simulink model "harness"  (R2024b)
settings: Solver=ode45  StartTime=0.0  StopTime=100  FixedStep=1/10  RelTol=1e-3
InitFcn:
  | init_fn()
undefined symbols (not defined in the file): sigbuilder_block
libraries: simulink x9
settings Model: PacingRate=10  Creator=Jacopo Sini  LastModifiedBy=aayan
settings OptimizationCC: ReuseModelBlockBuffer=off
settings DebuggingCC: UnconnectedInputMsg=warning  UnconnectedOutputMsg=warning  UnconnectedLineMsg=warning
settings ModelReferenceCC: EnableRefExpFcnMdlSchedulingChecks=on
settings RTWCC: GPUComputeCapability=3.5  DLArmComputeVersion=19.05

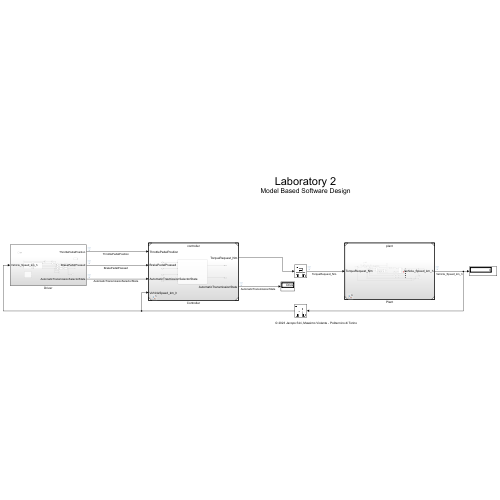
[thumbnail: Simulink's stored preview of the top-level diagram]
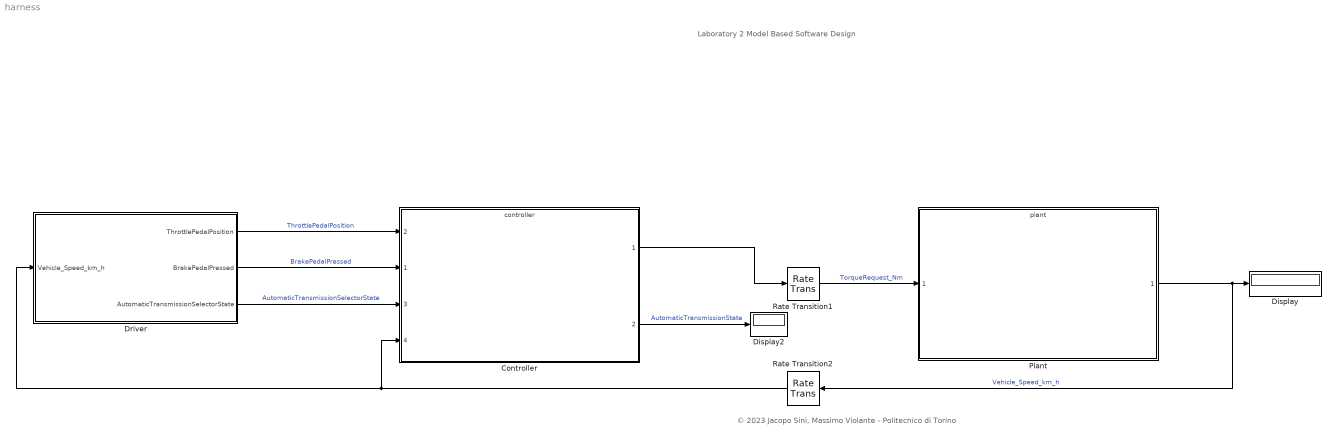
== system harness ==
  note: © 2023 Jacopo Sini, Massimo Violante - Politecnico di Torino
  note: Laboratory 2
      | Model Based Software Design
  Controller : ModelReference  ModelNameDialog=controller  SimulationMode=Normal  ModelReferenceVersion=7.15
      settings: PortSchema="{\"entries\":[{\"content\":{\"sides\":[{\"content\":{\"connectorIds\":[\"In2\",\"In1\",\"In3\",\"In4\"]},\"type\":\"ConnectorPlacement.EquallySpacedRectSide\",\"uuid\":\"5e260b81-e1ce-497c-8572-ac5c2182ee27\"},{\"content\":{\"connectorIds\":[\"Out1\",\"Out2\"],\"side\":\"RIGHT\"},\"type\":\"ConnectorPlacement.EquallySpacedRectSide\",\"uuid\":\"4325f63c-e453-4c79-ab01-1476da99aa25\"},{\"content\":{\"connectorIds\":[],\"side\":\"TOP\"},\"type\":\"ConnectorPlacement.EquallySpacedRectSide\",\"uuid\":\"dba88bac-0f95-4a98-ba3b-c40df5616f56\"}]},\"type\":\"ConnectorPlacement.EquallySpacedConnector\",\"uuid\":\"6943e10d-f3b0-4fd8-a142-b6b49e651f90\"}],\"packageUris\":[\"http://schema.mathworks.com/mf0/Connector/R2020b\"],\"version\":\"1.0\"}"
  Display : Display
  Display2 : Display
  Driver : Subsystem
  Plant : ModelReference  ModelNameDialog=plant  SimulationMode=Normal  ModelReferenceVersion=3.19
  Rate Transition1 : RateTransition
  Rate Transition2 : RateTransition
  wires:
  Plant/1 -> Rate Transition2/1, Display/1  "Vehicle_Speed_km_h"
  Controller/1 -> Rate Transition1/1
  Rate Transition2/1 -> Driver/1(Vehicle_Speed_km_h), Controller/4
  Controller/2 -> Display2/1  "AutomaticTransmissionState"
  Rate Transition1/1 -> Plant/1  "TorqueRequest_Nm"
  Driver/1(ThrottlePedalPosition) -> Controller/2  "ThrottlePedalPosition"
  Driver/2(BrakePedalPressed) -> Controller/1  "BrakePedalPressed"
  Driver/3(AutomaticTransmissionSelectorState) -> Controller/3  "AutomaticTransmissionSelectorState"

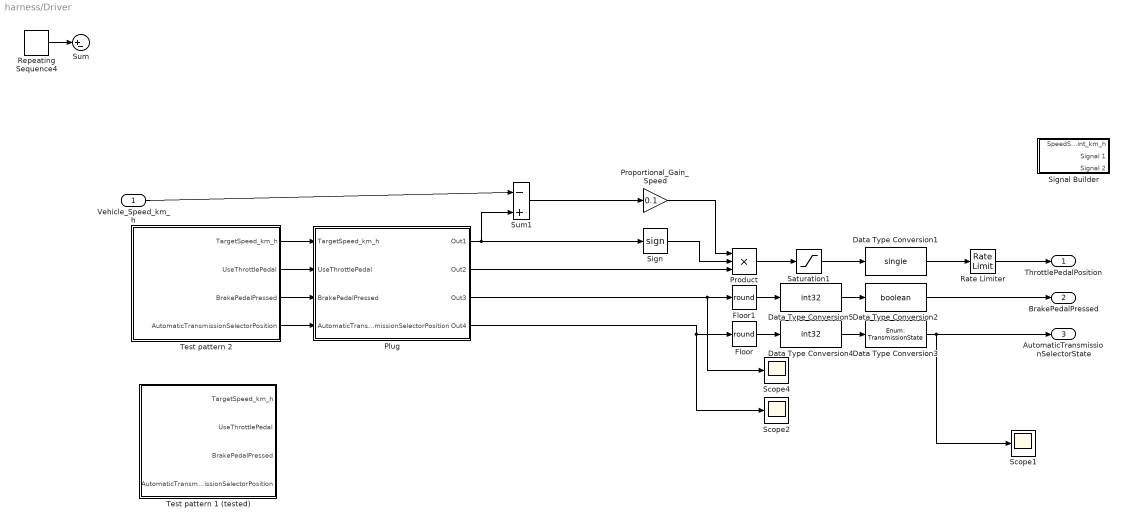
== system harness/Driver ==
  Vehicle_Speed_km_h : Inport
  Data Type Conversion1 : DataTypeConversion  OutDataTypeStr=single  SaturateOnIntegerOverflow=off  RndMeth=Floor  LockScale=on
  Data Type Conversion2 : DataTypeConversion  OutDataTypeStr=boolean  SaturateOnIntegerOverflow=off  RndMeth=Floor  LockScale=on
  Data Type Conversion3 : DataTypeConversion  OutDataTypeStr=Enum: TransmissionState  SaturateOnIntegerOverflow=off  RndMeth=Floor  LockScale=on
  Data Type Conversion4 : DataTypeConversion  OutDataTypeStr=int32  SaturateOnIntegerOverflow=off  RndMeth=Floor  LockScale=on
  Data Type Conversion5 : DataTypeConversion  OutDataTypeStr=int32  SaturateOnIntegerOverflow=off  RndMeth=Floor  LockScale=on
  Floor : Rounding  Operator=round
  Floor1 : Rounding  Operator=round
  Plug : Subsystem
  Product : Product  Inputs=3
  Proportional_Gain_Speed : Gain  Gain=0.1
  Rate Limiter : RateLimiter  RisingSlewLimit=0.5  SampleTimeMode=inherited
  Repeating Sequence4 : simulink/Sources/Repeating Sequence  rep_seq_t=[0 10 500]  rep_seq_y=[10 0 0]
  Saturation1 : Saturate  UpperLimit=1  LowerLimit=0
  Scope1 : Scope
  Scope2 : Scope
  Scope4 : Scope
  Sign : Signum
  Signal Builder : Subsystem  Tag=STV Subsys  LoadFcn=sigbuilder_block('load');  StartFcn=sigbuilder_block('start');  StopFcn=sigbuilder_block('stop');  ClipboardFcn=sigbuilder_block('clipboard');  mask(Sigbuilder block){tuvar=[0:10]}
      mask help: Simulink:masks:SigbuilderBlock_MD
      mask init:
      | if ~strcmp(get_param(bdroot(gcbh),'SimulationStatus'),'stopped') tuvar = sigbuilder_block('maskInit'); end
      settings: CopyFcn=sigbuilder_block('copy');  DeleteFcn=sigbuilder_block('delete');  ModelCloseFcn=sigbuilder_block('modelClose');  PreSaveFcn=sigbuilder_block('preSave');  PauseFcn=sigbuilder_block('pause');  ContinueFcn=sigbuilder_block('continue');  NameChangeFcn=sigbuilder_block('namechange');  OpenFcn=sigbuilder_block('open',[0 84 2240 1072 ]);  CloseFcn=sigbuilder_block('close');
      mask Display: plot(0, 0, 100, 100,[2, 2, 32, 32, 2], [68, 8, 8, 68, 68],[32, 2], [38, 38], [32, 19, 2],[53, 60, 44], [32, 17, 17, 2],[16, 16, 31, 31]);txt = getActiveGroup(gcbh);text(2, 100, txt,'verticalAlignment', 'top');
  Sum : Sum  Inputs=|+-
  Sum1 : Sum  Inputs=|-+
  Test pattern 1 (tested) : Subsystem
  Test pattern 2 : Subsystem
  ThrottlePedalPosition : Outport
  BrakePedalPressed : Outport  Port=2
  AutomaticTransmissionSelectorState : Outport  Port=3  OutDataTypeStr=Enum: TransmissionState
  wires:
  Data Type Conversion1/1 -> Rate Limiter/1
  Data Type Conversion2/1 -> BrakePedalPressed/1
  Data Type Conversion3/1 -> AutomaticTransmissionSelectorState/1, Scope1/1
  Floor/1 -> Data Type Conversion4/1
  Data Type Conversion4/1 -> Data Type Conversion3/1
  Floor1/1 -> Data Type Conversion5/1
  Data Type Conversion5/1 -> Data Type Conversion2/1
  Product/1 -> Saturation1/1
  Sum1/1 -> Proportional_Gain_Speed/1
  Sign/1 -> Product/2
  Saturation1/1 -> Data Type Conversion1/1
  Rate Limiter/1 -> ThrottlePedalPosition/1
  Repeating Sequence4/1 -> Sum/1
  Vehicle_Speed_km_h/1 -> Sum1/1
  Proportional_Gain_Speed/1 -> Product/1
  Plug/1(Out1) -> Sum1/2, Sign/1
  Plug/3(Out3) -> Scope4/1, Floor1/1
  Plug/4(Out4) -> Scope2/1, Floor/1
  Plug/2(Out2) -> Product/3
  Test pattern 2/1(TargetSpeed_km_h) -> Plug/1(TargetSpeed_km_h)
  Test pattern 2/2(UseThrottlePedal) -> Plug/2(UseThrottlePedal)
  Test pattern 2/3(BrakePedalPressed) -> Plug/3(BrakePedalPressed)
  Test pattern 2/4(AutomaticTransmissionSelectorPosition) -> Plug/4(AutomaticTransmissionSelectorPosition)

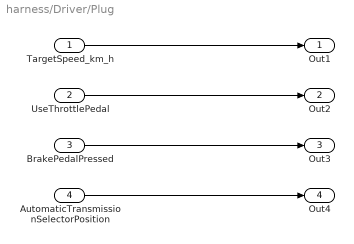
== system harness/Driver/Plug ==
  TargetSpeed_km_h : Inport
  UseThrottlePedal : Inport  Port=2
  BrakePedalPressed : Inport  Port=3
  AutomaticTransmissionSelectorPosition : Inport  Port=4
  Out1 : Outport
  Out2 : Outport  Port=2
  Out3 : Outport  Port=3
  Out4 : Outport  Port=4
  wires:
  TargetSpeed_km_h/1 -> Out1/1
  UseThrottlePedal/1 -> Out2/1
  BrakePedalPressed/1 -> Out3/1
  AutomaticTransmissionSelectorPosition/1 -> Out4/1

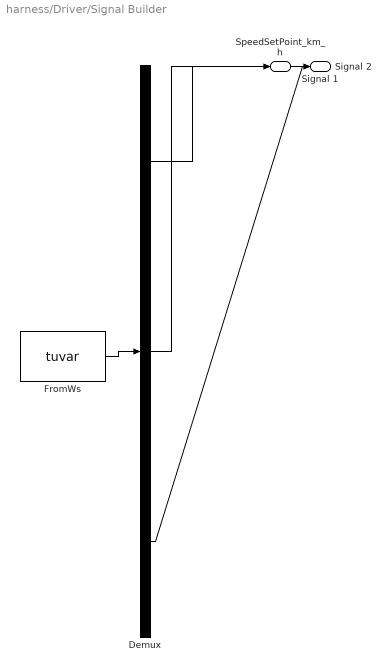
== system harness/Driver/Signal Builder ==
  Demux : Demux  Tag=STV Demux  Outputs=3
      settings: DisplayOption=none
  FromWs : FromWorkspace  Tag=STV FromWs  VariableName=tuvar
      SigBuilderData=|
      | common.afterFinalStr = 'Extrapolate'
      | common.sampleTime = 0
      | dataSet.timeRange = [0 500]
      | dataSet.name = 'Group 1'
      | sbobj.Groups.Name = 'Group 1'
      | sbobj.Groups.Signals(1).Name = 'SpeedSetPoint_km_h'
      | sbobj.Groups.Signals(1).XData = [0 2.165 2.165 6 6 500]
      | sbobj.Groups.Signals(1).YData = [0 0 1 1 0 0]
      | sbobj.Groups.Signals(2).Name = 'Signal 1'
      | sbobj.Groups.Signals(2).XData = [0 0.5 0.5 1 1 1.5 1.5 2 2 2.5 2.5 3 ... (2000 elements, 1x2000)]
      | sbobj.Groups.Signals(2).YData = [2 2 0 0 2 2 0 0 2 2 0 0 ... (2000 elements, 1x2000)]
      | sbobj.Groups.Signals(3).Name = 'Signal 2'
      | sbobj.Groups.Signals(3).XData = [0 250 250 500]
      | sbobj.Groups.Signals(3).YData = [0 0 1 1]
      | sbobj.Groups.TimeRange = [0 500]
  SpeedSetPoint_km_h : Outport  Tag=STV Outport
  Signal 1 : Outport  Tag=STV Outport  Port=2
  Signal 2 : Outport  Tag=STV Outport  Port=3
  wires:
  Demux/1 -> SpeedSetPoint_km_h/1
  FromWs/1 -> Demux/1
  Demux/2 -> Signal 1/1
  Demux/3 -> Signal 2/1

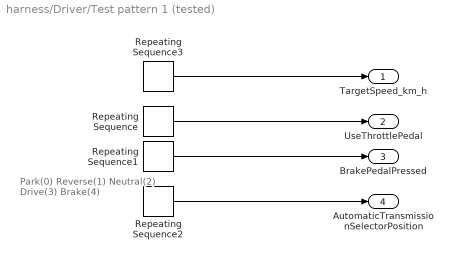
== system harness/Driver/Test pattern 1 (tested) ==
  note: Park(0)
      | Reverse(1)
      | Neutral(2)
      | Drive(3)
      | Brake(4)
  Repeating Sequence : simulink/Sources/Repeating Sequence  rep_seq_t=[0 3.9 4 500]  rep_seq_y=[0 0 1 1]
  Repeating Sequence1 : simulink/Sources/Repeating Sequence  rep_seq_t=[0 2.999 3 49.9 50.0 52.0 52.1 500]  rep_seq_y=[1 1 0 0 1 1 0 0]
  Repeating Sequence2 : simulink/Sources/Repeating Sequence  rep_seq_t=[0 1.999 2 10 49.9 50.0 500]  rep_seq_y=[0 0 4 4 4 1 1]
  Repeating Sequence3 : simulink/Sources/Repeating Sequence  rep_seq_t=[0 3.9 4 29.9 30 39.9 40 52.9 53 500]  rep_seq_y=[0 0 90 90 60 60 0 0 -20 -20]
  TargetSpeed_km_h : Outport
  UseThrottlePedal : Outport  Port=2
  BrakePedalPressed : Outport  Port=3
  AutomaticTransmissionSelectorPosition : Outport  Port=4
  wires:
  Repeating Sequence2/1 -> AutomaticTransmissionSelectorPosition/1
  Repeating Sequence/1 -> UseThrottlePedal/1
  Repeating Sequence1/1 -> BrakePedalPressed/1
  Repeating Sequence3/1 -> TargetSpeed_km_h/1

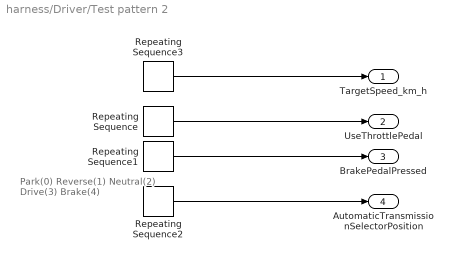
== system harness/Driver/Test pattern 2 ==
  note: Park(0)
      | Reverse(1)
      | Neutral(2)
      | Drive(3)
      | Brake(4)
  Repeating Sequence : simulink/Sources/Repeating Sequence  rep_seq_t=[0 3.9 4 500]  rep_seq_y=[0 0 1 1]
  Repeating Sequence1 : simulink/Sources/Repeating Sequence  rep_seq_t=[0 2.999 3 49.9 80.0 82.0 92.1 500]  rep_seq_y=[1 1 0 0 1 1 0 0]
  Repeating Sequence2 : simulink/Sources/Repeating Sequence  rep_seq_t=[0 1.999 2 10 79.9 80.0 500]  rep_seq_y=[0 0 4 4 4 1 1]
  Repeating Sequence3 : simulink/Sources/Repeating Sequence  rep_seq_t=[0 3.9 4 29.9 30 39.9 40 82.9 83 500]  rep_seq_y=[0 0 90 90 60 60 0 0 -20 -20]
  TargetSpeed_km_h : Outport
  UseThrottlePedal : Outport  Port=2
  BrakePedalPressed : Outport  Port=3
  AutomaticTransmissionSelectorPosition : Outport  Port=4
  wires:
  Repeating Sequence2/1 -> AutomaticTransmissionSelectorPosition/1
  Repeating Sequence/1 -> UseThrottlePedal/1
  Repeating Sequence1/1 -> BrakePedalPressed/1
  Repeating Sequence3/1 -> TargetSpeed_km_h/1
